simulink model "TwoLinkRobotCL_OpFbHpf"  (R2018b)
settings: Solver=VariableStepAuto  StartTime=0.0  StopTime=5  RelTol=1e-3
values from neighbouring files (symbols this model uses):
  DeltaSim =     [RandomDelta.mat]
  Hpf = ss(-1/tauHpf,-1/tauHpf,1/tauHpf,1/tauHpf)    [twoLinkRobot_OpFb.m]
  KSfb = -Klqr    [twoLinkRobot_LQR.m]    (also in twoLinkRobot_MonteCarloDisturbancePlot.m; twoLinkRobot_OpFb.m)
libraries: ltvlib x4
settings Model: Creator=pjseiler  LastModifiedBy=Jyot Buch
settings SFSimCC: SimUseLocalCustomCode=off
settings RTWCC: RTWUseLocalCustomCode=off
settings CodeAppCC: StateflowObjectComments=on

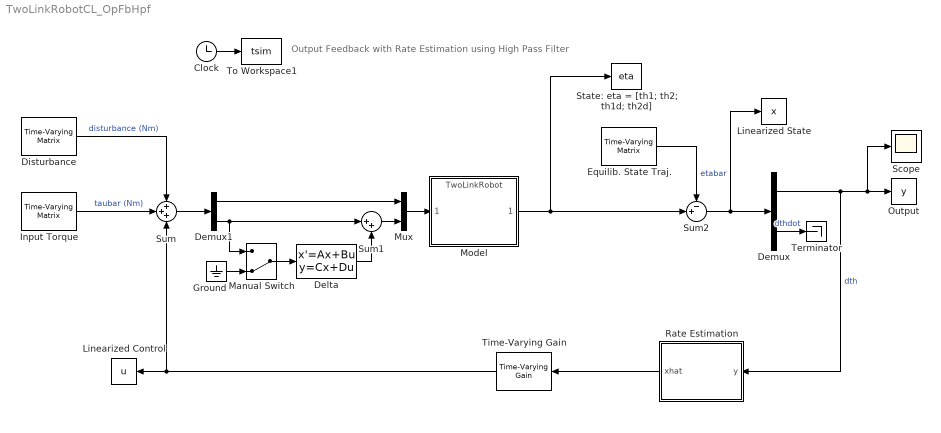
== system TwoLinkRobotCL_OpFbHpf ==
  note: Output Feedback with Rate Estimation using High Pass Filter
  Clock : Clock
  Delta : StateSpace  A=DeltaSim.A  B=DeltaSim.B  C=DeltaSim.C  D=DeltaSim.D  InitialCondition=0
  Demux : Demux  Outputs=[2,2]
  Demux1 : Demux  Outputs=2
  Disturbance : ltvlib/Time-Varying Matrix  M=d  vec1D=on
      settings: SourceProductName=Linear Time-Varying Systems Toolbox
  Equilib. State Traj. : ltvlib/Time-Varying Matrix  M=etabar  vec1D=on
      settings: SourceProductName=Linear Time-Varying Systems Toolbox
  Ground : Ground
  Input Torque : ltvlib/Time-Varying Matrix  M=taubar  vec1D=on
      settings: SourceProductName=Linear Time-Varying Systems Toolbox
  Linearized Control : ToWorkspace  VariableName=u  SampleTime=-1
  Linearized State : ToWorkspace  VariableName=x  SampleTime=-1
  Manual Switch : ManualSwitch  CurrentSetting=0
  Model : ModelReference  ModelNameDialog=TwoLinkRobot.slx  SimulationMode=Normal  ModelReferenceVersion=1.4
  Mux : Mux  Inputs=2
  Output : ToWorkspace  VariableName=y  SampleTime=-1
  Rate Estimation : Subsystem
  Scope : Scope
  State: eta = [th1; th2; th1d; th2d] : ToWorkspace  VariableName=eta  SampleTime=-1
  Sum : Sum  Inputs=+++
  Sum1 : Sum  Inputs=|++
  Sum2 : Sum  Inputs=-+|
  Terminator : Terminator
  Time-Varying Gain : ltvlib/Time-Varying Gain  K=KSfb
      settings: SourceProductName=Linear Time-Varying Systems Toolbox
  To Workspace1 : ToWorkspace  VariableName=tsim  SampleTime=-1
  wires:
  Clock/1 -> To Workspace1/1
  Disturbance/1 -> Sum/1  "disturbance (Nm)"
  Model/1 -> State: eta = [th1; th2; th1d; th2d]/1, Sum2/2
  Equilib. State Traj./1 -> Sum2/1  "etabar"
  Sum2/1 -> Demux/1, Linearized State/1
  Time-Varying Gain/1 -> Sum/3, Linearized Control/1
  Input Torque/1 -> Sum/2  "taubar (Nm)"
  Demux/2 -> Terminator/1  "dthdot"
  Demux/1 -> Scope/1, Output/1, Rate Estimation/1(y)  "dth"
  Rate Estimation/1(xhat) -> Time-Varying Gain/1
  Demux1/2 -> Sum1/1, Manual Switch/1
  Ground/1 -> Manual Switch/2
  Manual Switch/1 -> Delta/1
  Delta/1 -> Sum1/2
  Demux1/1 -> Mux/1
  Sum/1 -> Demux1/1
  Sum1/1 -> Mux/2
  Mux/1 -> Model/1

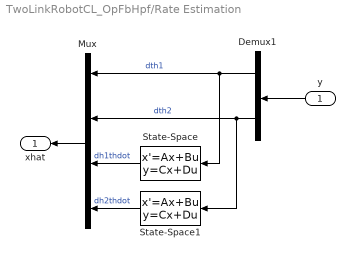
== system TwoLinkRobotCL_OpFbHpf/Rate Estimation ==
  y : Inport
  Demux1 : Demux  Outputs=2
  Mux : Mux
  State-Space : StateSpace  A=Hpf.A  B=Hpf.B  C=Hpf.C  D=Hpf.D  InitialCondition=0
  State-Space1 : StateSpace  A=Hpf.A  B=Hpf.B  C=Hpf.C  D=Hpf.D  InitialCondition=0
  xhat : Outport
  wires:
  State-Space/1 -> Mux/3  "dh1thdot"
  State-Space1/1 -> Mux/4  "dh2thdot"
  y/1 -> Demux1/1
  Demux1/1 -> Mux/1, State-Space/1  "dth1"
  Demux1/2 -> State-Space1/1, Mux/2  "dth2"
  Mux/1 -> xhat/1
